simulink model "model"  (R2014a)
(part 2 of 2)

      settings: AttributesFormatString=|
      | %<ID>
      | %<Vbase>V
      | %<VLF>pu
      | %<angleLF>deg.
      | %<Name>
  bus68 : powerlib/Measurements/Load Flow Bus  LConnTagsString=a  ID=bus68  Vbase=345000  Vref=1  Vangle=0  VLF=1  angleLF=0
      settings: AttributesFormatString=|
      | %<ID>
      | %<Vbase>V
      | %<VLF>pu
      | %<angleLF>deg.
      | %<Name>
  bus69 : powerlib/Measurements/Load Flow Bus  LConnTagsString=a  ID=bus69  Vbase=345000  Vref=1  Vangle=0  VLF=1  angleLF=0
      settings: AttributesFormatString=|
      | %<ID>
      | %<Vbase>V
      | %<VLF>pu
      | %<angleLF>deg.
      | %<Name>
  bus7 : powerlib/Measurements/Load Flow Bus  LConnTagsString=a  ID=bus7  Vbase=154000  Vref=1  Vangle=0  VLF=1  angleLF=0
      settings: AttributesFormatString=|
      | %<ID>
      | %<Vbase>V
      | %<VLF>pu
      | %<angleLF>deg.
      | %<Name>
  bus70 : powerlib/Measurements/Load Flow Bus  LConnTagsString=a  ID=bus70  Vbase=345000  Vref=1  Vangle=0  VLF=1  angleLF=0
      settings: AttributesFormatString=|
      | %<ID>
      | %<Vbase>V
      | %<VLF>pu
      | %<angleLF>deg.
      | %<Name>
  bus71 : powerlib/Measurements/Load Flow Bus  LConnTagsString=a  ID=bus71  Vbase=345000  Vref=1  Vangle=0  VLF=1  angleLF=0
      settings: AttributesFormatString=|
      | %<ID>
      | %<Vbase>V
      | %<VLF>pu
      | %<angleLF>deg.
      | %<Name>
  bus72 : powerlib/Measurements/Load Flow Bus  LConnTagsString=a  ID=bus72  Vbase=345000  Vref=1  Vangle=0  VLF=1  angleLF=0
      settings: AttributesFormatString=|
      | %<ID>
      | %<Vbase>V
      | %<VLF>pu
      | %<angleLF>deg.
      | %<Name>
  bus73 : powerlib/Measurements/Load Flow Bus  LConnTagsString=a  ID=bus73  Vbase=345000  Vref=1  Vangle=0  VLF=1  angleLF=0
      settings: AttributesFormatString=|
      | %<ID>
      | %<Vbase>V
      | %<VLF>pu
      | %<angleLF>deg.
      | %<Name>
  bus74 : powerlib/Measurements/Load Flow Bus  LConnTagsString=a  ID=bus74  Vbase=345000  Vref=1  Vangle=0  VLF=1  angleLF=0
      settings: AttributesFormatString=|
      | %<ID>
      | %<Vbase>V
      | %<VLF>pu
      | %<angleLF>deg.
      | %<Name>
  bus75 : powerlib/Measurements/Load Flow Bus  LConnTagsString=a  ID=bus75  Vbase=345000  Vref=1  Vangle=0  VLF=1  angleLF=0
      settings: AttributesFormatString=|
      | %<ID>
      | %<Vbase>V
      | %<VLF>pu
      | %<angleLF>deg.
      | %<Name>
  bus76 : powerlib/Measurements/Load Flow Bus  LConnTagsString=a  ID=bus76  Vbase=345000  Vref=1  Vangle=0  VLF=1  angleLF=0
      settings: AttributesFormatString=|
      | %<ID>
      | %<Vbase>V
      | %<VLF>pu
      | %<angleLF>deg.
      | %<Name>
  bus77 : powerlib/Measurements/Load Flow Bus  LConnTagsString=a  ID=bus77  Vbase=345000  Vref=1  Vangle=0  VLF=1  angleLF=0
      settings: AttributesFormatString=|
      | %<ID>
      | %<Vbase>V
      | %<VLF>pu
      | %<angleLF>deg.
      | %<Name>
  bus78 : powerlib/Measurements/Load Flow Bus  LConnTagsString=a  ID=bus78  Vbase=345000  Vref=1  Vangle=0  VLF=1  angleLF=0
      settings: AttributesFormatString=|
      | %<ID>
      | %<Vbase>V
      | %<VLF>pu
      | %<angleLF>deg.
      | %<Name>
  bus79 : powerlib/Measurements/Load Flow Bus  LConnTagsString=a  ID=bus79  Vbase=345000  Vref=1  Vangle=0  VLF=1  angleLF=0
      settings: AttributesFormatString=|
      | %<ID>
      | %<Vbase>V
      | %<VLF>pu
      | %<angleLF>deg.
      | %<Name>
  bus8 : powerlib/Measurements/Load Flow Bus  LConnTagsString=a  ID=bus8  Vbase=154000  Vref=1  Vangle=0  VLF=1  angleLF=0
      settings: AttributesFormatString=|
      | %<ID>
      | %<Vbase>V
      | %<VLF>pu
      | %<angleLF>deg.
      | %<Name>
  bus80 : powerlib/Measurements/Load Flow Bus  LConnTagsString=a  ID=bus80  Vbase=345000  Vref=1  Vangle=0  VLF=1  angleLF=0
      settings: AttributesFormatString=|
      | %<ID>
      | %<Vbase>V
      | %<VLF>pu
      | %<angleLF>deg.
      | %<Name>
  bus81 : powerlib/Measurements/Load Flow Bus  LConnTagsString=a  ID=bus81  Vbase=345000  Vref=1  Vangle=0  VLF=1  angleLF=0
      settings: AttributesFormatString=|
      | %<ID>
      | %<Vbase>V
      | %<VLF>pu
      | %<angleLF>deg.
      | %<Name>
  bus82 : powerlib/Measurements/Load Flow Bus  LConnTagsString=a  ID=bus82  Vbase=345000  Vref=1  Vangle=0  VLF=1  angleLF=0
      settings: AttributesFormatString=|
      | %<ID>
      | %<Vbase>V
      | %<VLF>pu
      | %<angleLF>deg.
      | %<Name>
  bus83 : powerlib/Measurements/Load Flow Bus  LConnTagsString=a  ID=bus83  Vbase=345000  Vref=1  Vangle=0  VLF=1  angleLF=0
      settings: AttributesFormatString=|
      | %<ID>
      | %<Vbase>V
      | %<VLF>pu
      | %<angleLF>deg.
      | %<Name>
  bus84 : powerlib/Measurements/Load Flow Bus  LConnTagsString=a  ID=bus84  Vbase=345000  Vref=1  Vangle=0  VLF=1  angleLF=0
      settings: AttributesFormatString=|
      | %<ID>
      | %<Vbase>V
      | %<VLF>pu
      | %<angleLF>deg.
      | %<Name>
  bus85 : powerlib/Measurements/Load Flow Bus  LConnTagsString=a  ID=bus85  Vbase=345000  Vref=1  Vangle=0  VLF=1  angleLF=0
      settings: AttributesFormatString=|
      | %<ID>
      | %<Vbase>V
      | %<VLF>pu
      | %<angleLF>deg.
      | %<Name>
  bus86 : powerlib/Measurements/Load Flow Bus  LConnTagsString=a  ID=bus86  Vbase=345000  Vref=1  Vangle=0  VLF=1  angleLF=0
      settings: AttributesFormatString=|
      | %<ID>
      | %<Vbase>V
      | %<VLF>pu
      | %<angleLF>deg.
      | %<Name>
  bus87 : powerlib/Measurements/Load Flow Bus  LConnTagsString=a  ID=bus87  Vbase=345000  Vref=1  Vangle=0  VLF=1  angleLF=0
      settings: AttributesFormatString=|
      | %<ID>
      | %<Vbase>V
      | %<VLF>pu
      | %<angleLF>deg.
      | %<Name>
  bus88 : powerlib/Measurements/Load Flow Bus  LConnTagsString=a  ID=bus88  Vbase=345000  Vref=1  Vangle=0  VLF=1  angleLF=0
      settings: AttributesFormatString=|
      | %<ID>
      | %<Vbase>V
      | %<VLF>pu
      | %<angleLF>deg.
      | %<Name>
  bus89 : powerlib/Measurements/Load Flow Bus  LConnTagsString=a  ID=bus89  Vbase=345000  Vref=1  Vangle=0  VLF=1  angleLF=0
      settings: AttributesFormatString=|
      | %<ID>
      | %<Vbase>V
      | %<VLF>pu
      | %<angleLF>deg.
      | %<Name>
  bus9 : powerlib/Measurements/Load Flow Bus  LConnTagsString=a  ID=bus9  Vbase=154000  Vref=1  Vangle=0  VLF=1  angleLF=0
      settings: AttributesFormatString=|
      | %<ID>
      | %<Vbase>V
      | %<VLF>pu
      | %<angleLF>deg.
      | %<Name>
  bus90 : powerlib/Measurements/Load Flow Bus  LConnTagsString=a  ID=bus90  Vbase=345000  Vref=1  Vangle=0  VLF=1  angleLF=0
      settings: AttributesFormatString=|
      | %<ID>
      | %<Vbase>V
      | %<VLF>pu
      | %<angleLF>deg.
      | %<Name>
  bus91 : powerlib/Measurements/Load Flow Bus  LConnTagsString=a  ID=bus91  Vbase=345000  Vref=1  Vangle=0  VLF=1  angleLF=0
      settings: AttributesFormatString=|
      | %<ID>
      | %<Vbase>V
      | %<VLF>pu
      | %<angleLF>deg.
      | %<Name>
  bus92 : powerlib/Measurements/Load Flow Bus  LConnTagsString=a  ID=bus92  Vbase=345000  Vref=1  Vangle=0  VLF=1  angleLF=0
      settings: AttributesFormatString=|
      | %<ID>
      | %<Vbase>V
      | %<VLF>pu
      | %<angleLF>deg.
      | %<Name>
  bus93 : powerlib/Measurements/Load Flow Bus  LConnTagsString=a  ID=bus93  Vbase=345000  Vref=1  Vangle=0  VLF=1  angleLF=0
      settings: AttributesFormatString=|
      | %<ID>
      | %<Vbase>V
      | %<VLF>pu
      | %<angleLF>deg.
      | %<Name>
  bus94 : powerlib/Measurements/Load Flow Bus  LConnTagsString=a  ID=bus94  Vbase=345000  Vref=1  Vangle=0  VLF=1  angleLF=0
      settings: AttributesFormatString=|
      | %<ID>
      | %<Vbase>V
      | %<VLF>pu
      | %<angleLF>deg.
      | %<Name>
  bus95 : powerlib/Measurements/Load Flow Bus  LConnTagsString=a  ID=bus95  Vbase=345000  Vref=1  Vangle=0  VLF=1  angleLF=0
      settings: AttributesFormatString=|
      | %<ID>
      | %<Vbase>V
      | %<VLF>pu
      | %<angleLF>deg.
      | %<Name>
  bus96 : powerlib/Measurements/Load Flow Bus  LConnTagsString=a  ID=bus96  Vbase=345000  Vref=1  Vangle=0  VLF=1  angleLF=0
      settings: AttributesFormatString=|
      | %<ID>
      | %<Vbase>V
      | %<VLF>pu
      | %<angleLF>deg.
      | %<Name>
  bus97 : powerlib/Measurements/Load Flow Bus  LConnTagsString=a  ID=bus97  Vbase=345000  Vref=1  Vangle=0  VLF=1  angleLF=0
      settings: AttributesFormatString=|
      | %<ID>
      | %<Vbase>V
      | %<VLF>pu
      | %<angleLF>deg.
      | %<Name>
  bus98 : powerlib/Measurements/Load Flow Bus  LConnTagsString=a  ID=bus98  Vbase=345000  Vref=1  Vangle=0  VLF=1  angleLF=0
      settings: AttributesFormatString=|
      | %<ID>
      | %<Vbase>V
      | %<VLF>pu
      | %<angleLF>deg.
      | %<Name>
  bus99 : powerlib/Measurements/Load Flow Bus  LConnTagsString=a  ID=bus99  Vbase=345000  Vref=1  Vangle=0  VLF=1  angleLF=0
      settings: AttributesFormatString=|
      | %<ID>
      | %<Vbase>V
      | %<VLF>pu
      | %<angleLF>deg.
      | %<Name>
  powergui : powerlib/powergui  Priority=1  SimulationMode=Continuous  SolverType=Tustin  SampleTime=50e-6  frequency=60  SPID=off  DisableSnubberDevices=off  DisableRonSwitches=off  DisableVfSwitches=off  SwTol=0  Interpol=off  DisplayEquations=off  Ts=0  methode=off  frequencyindice=60  Pbase=100e6  ErrMax=1e-4  Iterations=50  UnitsV=kV  UnitsW=MW  FunctionMessages=off  echomessages=off  HookPort=off  EnableUseOfTLC=off  x0status=blocks  RestoreLinks=warning  ResistiveCurrentMeasurement=off  Frange=[0:2:500]  Ylog=off  Xlog=on  ShowGrid=off  save=off  variable=ZData  structure=0  ZoomFFT=off  StartTime=0.0  cycles=1  DisplayStyle=1  fundamental=60  FreqAxis=off  MaxFrequency=1000  frequencyindicesteady=1  RmsSteady=1  display=off
  connections:
  T_172009221_154000_/LConn1 -- _CN_172009221_154000_CN_119180549_154000/LConn1
  T_172009221_154000_/LConn2 -- _CN_172009221_154000_CN_119180549_154000/LConn2
  _CN_172009221_154000_CN_119180549_154000/LConn3 -- T_172009221_154000_/LConn3 -- bus1/LConn1
  T_119180549__/LConn1 -- _CN_172009221_154000_CN_119180549_154000/RConn1
  T_119180549__/LConn2 -- _CN_172009221_154000_CN_119180549_154000/RConn2
  _CN_172009221_154000_CN_119180549_154000/RConn3 -- T_119180549__/LConn3 -- bus2/LConn1
  _CN_310266400_154000_CN_312375473_154000/LConn1 -- T_310266400_345000_/RConn1 -- _CN_310266400_154000_CN_313654649_154000/LConn1 -- L_310266400/LConn1
  _CN_310266400_154000_CN_312375473_154000/LConn2 -- T_310266400_345000_/RConn2 -- _CN_310266400_154000_CN_313654649_154000/LConn2 -- L_310266400/LConn2
  _CN_310266400_154000_CN_312375473_154000/LConn3 -- T_310266400_345000_/RConn3 -- _CN_310266400_154000_CN_313654649_154000/LConn3 -- L_310266400/LConn3 -- bus3/LConn1
  _CN_310266400_154000_CN_312375473_154000/RConn1 -- T_312375473_154000_/LConn1 -- _CN_312375473_154000_CN_312375513_154000/LConn1 -- _CN_312375473_154000_CN_312375502_154000/LConn1
  _CN_310266400_154000_CN_312375473_154000/RConn2 -- T_312375473_154000_/LConn2 -- _CN_312375473_154000_CN_312375513_154000/LConn2 -- _CN_312375473_154000_CN_312375502_154000/LConn2
  _CN_310266400_154000_CN_312375473_154000/RConn3 -- T_312375473_154000_/LConn3 -- _CN_312375473_154000_CN_312375513_154000/LConn3 -- _CN_312375473_154000_CN_312375502_154000/LConn3 -- bus4/LConn1
  T_313654649_154000_/LConn1 -- _CN_310266400_154000_CN_313654649_154000/RConn1
  T_313654649_154000_/LConn2 -- _CN_310266400_154000_CN_313654649_154000/RConn2
  _CN_310266400_154000_CN_313654649_154000/RConn3 -- T_313654649_154000_/LConn3 -- bus5/LConn1
  _CN_180075042_154000_CN_168904645_154000/LConn1 -- T_180075042_154000_/LConn1 -- _CN_180075042_154000_CN_313283373_154000/LConn1
  _CN_180075042_154000_CN_168904645_154000/LConn2 -- T_180075042_154000_/LConn2 -- _CN_180075042_154000_CN_313283373_154000/LConn2
  _CN_180075042_154000_CN_168904645_154000/LConn3 -- T_180075042_154000_/LConn3 -- _CN_180075042_154000_CN_313283373_154000/LConn3 -- bus6/LConn1
  T_168904645__양양변전소/LConn1 -- _CN_180075042_154000_CN_168904645_154000/RConn1
  T_168904645__양양변전소/LConn2 -- _CN_180075042_154000_CN_168904645_154000/RConn2
  _CN_180075042_154000_CN_168904645_154000/RConn3 -- T_168904645__양양변전소/LConn3 -- bus7/LConn1
  T_313283373_154000_/LConn1 -- _CN_180075042_154000_CN_313283373_154000/RConn1
  T_313283373_154000_/LConn2 -- _CN_180075042_154000_CN_313283373_154000/RConn2
  _CN_180075042_154000_CN_313283373_154000/RConn3 -- T_313283373_154000_/LConn3 -- bus8/LConn1
  T_311068711_154000_/LConn1 -- _CN_311068711_154000_CN_205296347_154000/LConn1
  T_311068711_154000_/LConn2 -- _CN_311068711_154000_CN_205296347_154000/LConn2
  _CN_311068711_154000_CN_205296347_154000/LConn3 -- T_311068711_154000_/LConn3 -- bus9/LConn1
  _CN_311068711_154000_CN_205296347_154000/RConn1 -- T_205296347__/LConn1 -- _CN_308953870_154000_CN_205296347_154000/LConn1
  _CN_311068711_154000_CN_205296347_154000/RConn2 -- T_205296347__/LConn2 -- _CN_308953870_154000_CN_205296347_154000/LConn2
  _CN_311068711_154000_CN_205296347_154000/RConn3 -- T_205296347__/LConn3 -- _CN_308953870_154000_CN_205296347_154000/LConn3 -- bus10/LConn1
  T_311144496_154000_/LConn1 -- _CN_311144496_154000_CN_316124722_154000/LConn1
  T_311144496_154000_/LConn2 -- _CN_311144496_154000_CN_316124722_154000/LConn2
  _CN_311144496_154000_CN_316124722_154000/LConn3 -- T_311144496_154000_/LConn3 -- bus11/LConn1
  T_316124722_154000_/LConn1 -- _CN_311144496_154000_CN_316124722_154000/RConn1
  T_316124722_154000_/LConn2 -- _CN_311144496_154000_CN_316124722_154000/RConn2
  _CN_311144496_154000_CN_316124722_154000/RConn3 -- T_316124722_154000_/LConn3 -- bus12/LConn1
  _CN_310293553_154000_CN_313388404_154000/LConn1 -- T_310293553_345000_/RConn1 -- L_310293553/LConn1
  _CN_310293553_154000_CN_313388404_154000/LConn2 -- T_310293553_345000_/RConn2 -- L_310293553/LConn2
  _CN_310293553_154000_CN_313388404_154000/LConn3 -- T_310293553_345000_/RConn3 -- L_310293553/LConn3 -- bus13/LConn1
  _CN_310293553_154000_CN_313388404_154000/RConn1 -- T_313388404_154000_/LConn1 -- _CN_313388404_154000_CN_313388489_154000/LConn1
  _CN_310293553_154000_CN_313388404_154000/RConn2 -- T_313388404_154000_/LConn2 -- _CN_313388404_154000_CN_313388489_154000/LConn2
  _CN_310293553_154000_CN_313388404_154000/RConn3 -- T_313388404_154000_/LConn3 -- _CN_313388404_154000_CN_313388489_154000/LConn3 -- bus14/LConn1
  T_125840986__/LConn1 -- _CN_125840986_154000_CN_126047655_154000/LConn1
  T_125840986__/LConn2 -- _CN_125840986_154000_CN_126047655_154000/LConn2
  _CN_125840986_154000_CN_126047655_154000/LConn3 -- T_125840986__/LConn3 -- bus15/LConn1
  T_126047655__/LConn1 -- _CN_125840986_154000_CN_126047655_154000/RConn1
  T_126047655__/LConn2 -- _CN_125840986_154000_CN_126047655_154000/RConn2
  _CN_125840986_154000_CN_126047655_154000/RConn3 -- T_126047655__/LConn3 -- bus16/LConn1
  T_231045732__/LConn1 -- _CN_231045732_154000_CN_310574464_154000/LConn1
  T_231045732__/LConn2 -- _CN_231045732_154000_CN_310574464_154000/LConn2
  _CN_231045732_154000_CN_310574464_154000/LConn3 -- T_231045732__/LConn3 -- bus17/LConn1
  _CN_231045732_154000_CN_310574464_154000/RConn1 -- T_310574464__신진천_(Sin_Jincheon)/RConn1 -- _CN_308953870_154000_CN_310574464_154000/LConn1 -- L_310574464/LConn1
  _CN_231045732_154000_CN_310574464_154000/RConn2 -- T_310574464__신진천_(Sin_Jincheon)/RConn2 -- _CN_308953870_154000_CN_310574464_154000/LConn2 -- L_310574464/LConn2
  _CN_231045732_154000_CN_310574464_154000/RConn3 -- T_310574464__신진천_(Sin_Jincheon)/RConn3 -- _CN_308953870_154000_CN_310574464_154000/LConn3 -- L_310574464/LConn3 -- bus18/LConn1
  _CN_312297594_154000_CN_312297600_154000/LConn1 -- T_312297594_345000_신파주_(Sin_Paju)/RConn1 -- _CN_312297594_154000_CN_310963709_154000/LConn1 -- L_312297594/LConn1
  _CN_312297594_154000_CN_312297600_154000/LConn2 -- T_312297594_345000_신파주_(Sin_Paju)/RConn2 -- _CN_312297594_154000_CN_310963709_154000/LConn2 -- L_312297594/LConn2
  _CN_312297594_154000_CN_312297600_154000/LConn3 -- T_312297594_345000_신파주_(Sin_Paju)/RConn3 -- _CN_312297594_154000_CN_310963709_154000/LConn3 -- L_312297594/LConn3 -- bus19/LConn1
  T_312297600_154000_/LConn1 -- _CN_312297594_154000_CN_312297600_154000/RConn1
  T_312297600_154000_/LConn2 -- _CN_312297594_154000_CN_312297600_154000/RConn2
  _CN_312297594_154000_CN_312297600_154000/RConn3 -- T_312297600_154000_/LConn3 -- bus20/LConn1
  _CN_312297594_154000_CN_310963709_154000/RConn1 -- T_310963709__양주_(Yangju)/RConn1 -- L_310963709/LConn1
  _CN_312297594_154000_CN_310963709_154000/RConn2 -- T_310963709__양주_(Yangju)/RConn2 -- L_310963709/LConn2
  _CN_312297594_154000_CN_310963709_154000/RConn3 -- T_310963709__양주_(Yangju)/RConn3 -- L_310963709/LConn3 -- bus21/LConn1
  T_313247877_154000_/LConn1 -- _CN_313247877_154000_CN_313264823_154000/LConn1
  T_313247877_154000_/LConn2 -- _CN_313247877_154000_CN_313264823_154000/LConn2
  _CN_313247877_154000_CN_313264823_154000/LConn3 -- T_313247877_154000_/LConn3 -- bus22/LConn1
  T_313264823_154000_/LConn1 -- _CN_313247877_154000_CN_313264823_154000/RConn1
  T_313264823_154000_/LConn2 -- _CN_313247877_154000_CN_313264823_154000/RConn2
  _CN_313247877_154000_CN_313264823_154000/RConn3 -- T_313264823_154000_/LConn3 -- bus23/LConn1
  T_297601178_154000_/LConn1 -- _CN_297601178_154000_CN_297601183_154000/LConn1
  T_297601178_154000_/LConn2 -- _CN_297601178_154000_CN_297601183_154000/LConn2
  _CN_297601178_154000_CN_297601183_154000/LConn3 -- T_297601178_154000_/LConn3 -- bus24/LConn1
  _CN_297601178_154000_CN_297601183_154000/RConn1 -- T_297601183_154000_/LConn1 -- _CN_297601183_154000_CN_308765055_154000/LConn1 -- _CN_297601183_154000_CN_308765054_154000/LConn1
  _CN_297601178_154000_CN_297601183_154000/RConn2 -- T_297601183_154000_/LConn2 -- _CN_297601183_154000_CN_308765055_154000/LConn2 -- _CN_297601183_154000_CN_308765054_154000/LConn2
  _CN_297601178_154000_CN_297601183_154000/RConn3 -- T_297601183_154000_/LConn3 -- _CN_297601183_154000_CN_308765055_154000/LConn3 -- _CN_297601183_154000_CN_308765054_154000/LConn3 -- bus25/LConn1
  _CN_297601183_154000_CN_308765055_154000/RConn1 -- T_308765055__/RConn1 -- L_308765055/LConn1
  _CN_297601183_154000_CN_308765055_154000/RConn2 -- T_308765055__/RConn2 -- L_308765055/LConn2
  _CN_297601183_154000_CN_308765055_154000/RConn3 -- T_308765055__/RConn3 -- L_308765055/LConn3 -- bus26/LConn1
  _CN_297601183_154000_CN_308765054_154000/RConn1 -- T_308765054_345000_/LConn1 -- _CN_313355118_154000_CN_308765054_154000/LConn1
  _CN_297601183_154000_CN_308765054_154000/RConn2 -- T_308765054_345000_/LConn2 -- _CN_313355118_154000_CN_308765054_154000/LConn2
  _CN_297601183_154000_CN_308765054_154000/RConn3 -- T_308765054_345000_/LConn3 -- _CN_313355118_154000_CN_308765054_154000/LConn3 -- bus27/LConn1
  _CN_310065312_154000_CN_313280968_154000/LConn1 -- T_310065312__/RConn1 -- _CN_310065312_154000_CN_312319437_154000/LConn1 -- L_310065312/LConn1
  _CN_310065312_154000_CN_313280968_154000/LConn2 -- T_310065312__/RConn2 -- _CN_310065312_154000_CN_312319437_154000/LConn2 -- L_310065312/LConn2
  _CN_310065312_154000_CN_313280968_154000/LConn3 -- T_310065312__/RConn3 -- _CN_310065312_154000_CN_312319437_154000/LConn3 -- L_310065312/LConn3 -- bus28/LConn1
  T_313280968_154000_/LConn1 -- _CN_310065312_154000_CN_313280968_154000/RConn1
  T_313280968_154000_/LConn2 -- _CN_310065312_154000_CN_313280968_154000/RConn2
  _CN_310065312_154000_CN_313280968_154000/RConn3 -- T_313280968_154000_/LConn3 -- bus29/LConn1
  T_312319437_154000_/LConn1 -- _CN_310065312_154000_CN_312319437_154000/RConn1
  T_312319437_154000_/LConn2 -- _CN_310065312_154000_CN_312319437_154000/RConn2
  _CN_310065312_154000_CN_312319437_154000/RConn3 -- T_312319437_154000_/LConn3 -- bus30/LConn1
  _CN_310421552_154000_CN_312319401_154000/LConn1 -- T_310421552__/RConn1 -- _CN_310421552_154000_CN_312319351_154000/LConn1 -- L_310421552/LConn1
  _CN_310421552_154000_CN_312319401_154000/LConn2 -- T_310421552__/RConn2 -- _CN_310421552_154000_CN_312319351_154000/LConn2 -- L_310421552/LConn2
  _CN_310421552_154000_CN_312319401_154000/LConn3 -- T_310421552__/RConn3 -- _CN_310421552_154000_CN_312319351_154000/LConn3 -- L_310421552/LConn3 -- bus31/LConn1
  T_312319401__/LConn1 -- _CN_310421552_154000_CN_312319401_154000/RConn1
  T_312319401__/LConn2 -- _CN_310421552_154000_CN_312319401_154000/RConn2
  _CN_310421552_154000_CN_312319401_154000/RConn3 -- T_312319401__/LConn3 -- bus32/LConn1
  T_312319351_154000_/LConn1 -- _CN_310421552_154000_CN_312319351_154000/RConn1
  T_312319351_154000_/LConn2 -- _CN_310421552_154000_CN_312319351_154000/RConn2
  _CN_310421552_154000_CN_312319351_154000/RConn3 -- T_312319351_154000_/LConn3 -- bus33/LConn1
  _CN_312375473_154000_CN_312375513_154000/RConn1 -- T_312375513_154000_/LConn1 -- _CN_312375513_154000_CN_312375515_154000/LConn1 -- _CN_312375513_154000_CN_308770040_154000/LConn1
  _CN_312375473_154000_CN_312375513_154000/RConn2 -- T_312375513_154000_/LConn2 -- _CN_312375513_154000_CN_312375515_154000/LConn2 -- _CN_312375513_154000_CN_308770040_154000/LConn2
  _CN_312375473_154000_CN_312375513_154000/RConn3 -- T_312375513_154000_/LConn3 -- _CN_312375513_154000_CN_312375515_154000/LConn3 -- _CN_312375513_154000_CN_308770040_154000/LConn3 -- bus34/LConn1
  T_312375502_154000_/LConn1 -- _CN_312375473_154000_CN_312375502_154000/RConn1
  T_312375502_154000_/LConn2 -- _CN_312375473_154000_CN_312375502_154000/RConn2
  _CN_312375473_154000_CN_312375502_154000/RConn3 -- T_312375502_154000_/LConn3 -- bus35/LConn1
  _CN_313264824_154000_CN_308953870_154000/LConn1 -- T_313264824_154000_/LConn1 -- _CN_313264824_154000_CN_371952375_154000/LConn1
  _CN_313264824_154000_CN_308953870_154000/LConn2 -- T_313264824_154000_/LConn2 -- _CN_313264824_154000_CN_371952375_154000/LConn2
  _CN_313264824_154000_CN_308953870_154000/LConn3 -- T_313264824_154000_/LConn3 -- _CN_313264824_154000_CN_371952375_154000/LConn3 -- bus36/LConn1
  _CN_313264824_154000_CN_308953870_154000/RConn1 -- T_308953870__신진천_(Sin_Jincheon)/LConn1 -- _CN_308953870_154000_CN_310574464_154000/RConn1 -- _CN_308953870_154000_CN_205296347_154000/RConn1
  _CN_313264824_154000_CN_308953870_154000/RConn2 -- T_308953870__신진천_(Sin_Jincheon)/LConn2 -- _CN_308953870_154000_CN_310574464_154000/RConn2 -- _CN_308953870_154000_CN_205296347_154000/RConn2
  _CN_313264824_154000_CN_308953870_154000/RConn3 -- T_308953870__신진천_(Sin_Jincheon)/LConn3 -- _CN_308953870_154000_CN_310574464_154000/RConn3 -- _CN_308953870_154000_CN_205296347_154000/RConn3 -- bus37/LConn1
  T_371952375__/LConn1 -- _CN_313264824_154000_CN_371952375_154000/RConn1
  T_371952375__/LConn2 -- _CN_313264824_154000_CN_371952375_154000/RConn2
  _CN_313264824_154000_CN_371952375_154000/RConn3 -- T_371952375__/LConn3 -- bus38/LConn1
  T_372869919_154000_/LConn1 -- _CN_372869919_154000_CN_310226151_154000/LConn1
  T_372869919_154000_/LConn2 -- _CN_372869919_154000_CN_310226151_154000/LConn2
  _CN_372869919_154000_CN_310226151_154000/LConn3 -- T_372869919_154000_/LConn3 -- bus39/LConn1
  _CN_372869919_154000_CN_310226151_154000/RConn1 -- T_310226151_345000_신광주_(Sin_Gwangju)/RConn1 -- L_310226151/LConn1
  _CN_372869919_154000_CN_310226151_154000/RConn2 -- T_310226151_345000_신광주_(Sin_Gwangju)/RConn2 -- L_310226151/LConn2
  _CN_372869919_154000_CN_310226151_154000/RConn3 -- T_310226151_345000_신광주_(Sin_Gwangju)/RConn3 -- L_310226151/LConn3 -- bus40/LConn1
  _CN_312375499_154000_CN_312375501_154000/LConn1 -- T_312375499_154000_/LConn1 -- _CN_312375499_154000_CN_308770040_154000/LConn1
  _CN_312375499_154000_CN_312375501_154000/LConn2 -- T_312375499_154000_/LConn2 -- _CN_312375499_154000_CN_308770040_154000/LConn2
  _CN_312375499_154000_CN_312375501_154000/LConn3 -- T_312375499_154000_/LConn3 -- _CN_312375499_154000_CN_308770040_154000/LConn3 -- bus41/LConn1
  T_312375501_154000_/LConn1 -- _CN_312375499_154000_CN_312375501_154000/RConn1
  T_312375501_154000_/LConn2 -- _CN_312375499_154000_CN_312375501_154000/RConn2
  _CN_312375499_154000_CN_312375501_154000/RConn3 -- T_312375501_154000_/LConn3 -- bus42/LConn1
  _CN_312375499_154000_CN_308770040_154000/RConn1 -- T_308770040__고령_(Goryeong)/RConn1 -- _CN_312375513_154000_CN_308770040_154000/RConn1 -- L_308770040/LConn1
  _CN_312375499_154000_CN_308770040_154000/RConn2 -- T_308770040__고령_(Goryeong)/RConn2 -- _CN_312375513_154000_CN_308770040_154000/RConn2 -- L_308770040/LConn2
  _CN_312375499_154000_CN_308770040_154000/RConn3 -- T_308770040__고령_(Goryeong)/RConn3 -- _CN_312375513_154000_CN_308770040_154000/RConn3 -- L_308770040/LConn3 -- bus43/LConn1
  _CN_310395601_154000_CN_310395617_154000/LConn1 -- T_310395601_154000_/LConn1 -- _CN_310395601_154000_CN_310281776_154000/LConn1
  _CN_310395601_154000_CN_310395617_154000/LConn2 -- T_310395601_154000_/LConn2 -- _CN_310395601_154000_CN_310281776_154000/LConn2
  _CN_310395601_154000_CN_310395617_154000/LConn3 -- T_310395601_154000_/LConn3 -- _CN_310395601_154000_CN_310281776_154000/LConn3 -- bus44/LConn1
  T_310395617_154000_/LConn1 -- _CN_310395601_154000_CN_310395617_154000/RConn1
  T_310395617_154000_/LConn2 -- _CN_310395601_154000_CN_310395617_154000/RConn2
  _CN_310395601_154000_CN_310395617_154000/RConn3 -- T_310395617_154000_/LConn3 -- bus45/LConn1
  _CN_310395601_154000_CN_310281776_154000/RConn1 -- T_310281776_345000_신김해_(Sin_Gimhae)/RConn1 -- _CN_415837596_154000_CN_310281776_154000/LConn1 -- L_310281776/LConn1
  _CN_310395601_154000_CN_310281776_154000/RConn2 -- T_310281776_345000_신김해_(Sin_Gimhae)/RConn2 -- _CN_415837596_154000_CN_310281776_154000/LConn2 -- L_310281776/LConn2
  _CN_310395601_154000_CN_310281776_154000/RConn3 -- T_310281776_345000_신김해_(Sin_Gimhae)/RConn3 -- _CN_415837596_154000_CN_310281776_154000/LConn3 -- L_310281776/LConn3 -- bus46/LConn1
  T_312375515_154000_/LConn1 -- _CN_312375513_154000_CN_312375515_154000/RConn1
  T_312375515_154000_/LConn2 -- _CN_312375513_154000_CN_312375515_154000/RConn2
  _CN_312375513_154000_CN_312375515_154000/RConn3 -- T_312375515_154000_/LConn3 -- bus47/LConn1
  _CN_143609113_154000_CN_312424737_154000/LConn1 -- T_143609113_345000_/RConn1 -- L_143609113/LConn1
  _CN_143609113_154000_CN_312424737_154000/LConn2 -- T_143609113_345000_/RConn2 -- L_143609113/LConn2
  _CN_143609113_154000_CN_312424737_154000/LConn3 -- T_143609113_345000_/RConn3 -- L_143609113/LConn3 -- bus48/LConn1
  _CN_143609113_154000_CN_312424737_154000/RConn1 -- T_312424737_154000_/LConn1 -- _CN_312424737_154000_CN_313355100_154000/LConn1
  _CN_143609113_154000_CN_312424737_154000/RConn2 -- T_312424737_154000_/LConn2 -- _CN_312424737_154000_CN_313355100_154000/LConn2
  _CN_143609113_154000_CN_312424737_154000/RConn3 -- T_312424737_154000_/LConn3 -- _CN_312424737_154000_CN_313355100_154000/LConn3 -- bus49/LConn1
  T_312424733_154000_/LConn1 -- _CN_312424733_154000_CN_312424741_154000/LConn1
  T_312424733_154000_/LConn2 -- _CN_312424733_154000_CN_312424741_154000/LConn2
  _CN_312424733_154000_CN_312424741_154000/LConn3 -- T_312424733_154000_/LConn3 -- bus50/LConn1
  T_312424741_154000_/LConn1 -- _CN_312424733_154000_CN_312424741_154000/RConn1
  T_312424741_154000_/LConn2 -- _CN_312424733_154000_CN_312424741_154000/RConn2
  _CN_312424733_154000_CN_312424741_154000/RConn3 -- T_312424741_154000_/LConn3 -- bus51/LConn1
  T_313355100_154000_/LConn1 -- _CN_312424737_154000_CN_313355100_154000/RConn1
  T_313355100_154000_/LConn2 -- _CN_312424737_154000_CN_313355100_154000/RConn2
  _CN_312424737_154000_CN_313355100_154000/RConn3 -- T_313355100_154000_/LConn3 -- bus52/LConn1
  _CN_313355118_154000_CN_313355123_154000/LConn1 -- T_313355118_154000_/LConn1 -- _CN_313355118_154000_CN_308765054_154000/RConn1
  _CN_313355118_154000_CN_313355123_154000/LConn2 -- T_313355118_154000_/LConn2 -- _CN_313355118_154000_CN_308765054_154000/RConn2
  _CN_313355118_154000_CN_313355123_154000/LConn3 -- T_313355118_154000_/LConn3 -- _CN_313355118_154000_CN_308765054_154000/RConn3 -- bus53/LConn1
  T_313355123_154000_/LConn1 -- _CN_313355118_154000_CN_313355123_154000/RConn1
  T_313355123_154000_/LConn2 -- _CN_313355118_154000_CN_313355123_154000/RConn2
  _CN_313355118_154000_CN_313355123_154000/RConn3 -- T_313355123_154000_/LConn3 -- bus54/LConn1
  T_313388489_154000_/LConn1 -- _CN_313388404_154000_CN_313388489_154000/RConn1
  T_313388489_154000_/LConn2 -- _CN_313388404_154000_CN_313388489_154000/RConn2
  _CN_313388404_154000_CN_313388489_154000/RConn3 -- T_313388489_154000_/LConn3 -- bus55/LConn1
  T_312408983_154000_/LConn1 -- _CN_312408983_154000_CN_235152925_154000/LConn1
  T_312408983_154000_/LConn2 -- _CN_312408983_154000_CN_235152925_154000/LConn2
  _CN_312408983_154000_CN_235152925_154000/LConn3 -- T_312408983_154000_/LConn3 -- bus56/LConn1
  G_235152925_인천발전소/RConn1 -- _CN_312408983_154000_CN_235152925_154000/RConn1
  G_235152925_인천발전소/RConn2 -- _CN_312408983_154000_CN_235152925_154000/RConn2
  _CN_312408983_154000_CN_235152925_154000/RConn3 -- G_235152925_인천발전소/RConn3 -- bus57/LConn1
  T_415837596__/LConn1 -- _CN_415837596_154000_CN_310281776_154000/RConn1
  T_415837596__/LConn2 -- _CN_415837596_154000_CN_310281776_154000/RConn2
  _CN_415837596_154000_CN_310281776_154000/RConn3 -- T_415837596__/LConn3 -- bus58/LConn1
  T_312319393_154000_/LConn1 -- _CN_312319393_154000_CN_308711344_154000/LConn1
  T_312319393_154000_/LConn2 -- _CN_312319393_154000_CN_308711344_154000/LConn2
  _CN_312319393_154000_CN_308711344_154000/LConn3 -- T_312319393_154000_/LConn3 -- bus59/LConn1
  _CN_312319393_154000_CN_308711344_154000/RConn1 -- T_308711344_345000_서서울_(Seo_Seoul)/RConn1 -- L_308711344/LConn1
  _CN_312319393_154000_CN_308711344_154000/RConn2 -- T_308711344_345000_서서울_(Seo_Seoul)/RConn2 -- L_308711344/LConn2
  _CN_312319393_154000_CN_308711344_154000/RConn3 -- T_308711344_345000_서서울_(Seo_Seoul)/RConn3 -- L_308711344/LConn3 -- bus60/LConn1
  _CN_310574464_345000_CN_310065312_345000/LConn1 -- T_310574464__신진천_(Sin_Jincheon)/LConn1 -- _CN_310574464_345000_CN_308953834_345000/LConn1
  _CN_310574464_345000_CN_310065312_345000/LConn2 -- T_310574464__신진천_(Sin_Jincheon)/LConn2 -- _CN_310574464_345000_CN_308953834_345000/LConn2
  _CN_310574464_345000_CN_310065312_345000/LConn3 -- T_310574464__신진천_(Sin_Jincheon)/LConn3 -- _CN_310574464_345000_CN_308953834_345000/LConn3 -- bus61/LConn1
  _CN_310574464_345000_CN_310065312_345000/RConn1 -- T_310065312__/LConn1 -- _CN_310065312_345000_CN_156580308_345000/LConn1
  _CN_310574464_345000_CN_310065312_345000/RConn2 -- T_310065312__/LConn2 -- _CN_310065312_345000_CN_156580308_345000/LConn2
  _CN_310574464_345000_CN_310065312_345000/RConn3 -- T_310065312__/LConn3 -- _CN_310065312_345000_CN_156580308_345000/LConn3 -- bus62/LConn1
  _CN_310574464_345000_CN_308953834_345000/RConn1 -- T_308953834_345000_/LConn1 -- _CN_308953834_345000_CN_313247875_345000/LConn1
  _CN_310574464_345000_CN_308953834_345000/RConn2 -- T_308953834_345000_/LConn2 -- _CN_308953834_345000_CN_313247875_345000/LConn2
  _CN_310574464_345000_CN_308953834_345000/RConn3 -- T_308953834_345000_/LConn3 -- _CN_308953834_345000_CN_313247875_345000/LConn3 -- bus63/LConn1
  T_310574466_345000_/LConn1 -- _CN_310574466_345000_CN_143756950_345000/LConn1
  T_310574466_345000_/LConn2 -- _CN_310574466_345000_CN_143756950_345000/LConn2
  _CN_310574466_345000_CN_143756950_345000/LConn3 -- T_310574466_345000_/LConn3 -- bus64/LConn1
  _CN_310574466_345000_CN_143756950_345000/RConn1 -- T_143756950_345000_/LConn1 -- _CN_143756950_345000_CN_143609113_345000/LConn1
  _CN_310574466_345000_CN_143756950_345000/RConn2 -- T_143756950_345000_/LConn2 -- _CN_143756950_345000_CN_143609113_345000/LConn2
  _CN_310574466_345000_CN_143756950_345000/RConn3 -- T_143756950_345000_/LConn3 -- _CN_143756950_345000_CN_143609113_345000/LConn3 -- bus65/LConn1
  _CN_117614725_345000_CN_310266400_345000/LConn1 -- T_117614725__/LConn1 -- _CN_117614725_345000_CN_310281776_345000/LConn1
  _CN_117614725_345000_CN_310266400_345000/LConn2 -- T_117614725__/LConn2 -- _CN_117614725_345000_CN_310281776_345000/LConn2
  _CN_117614725_345000_CN_310266400_345000/LConn3 -- T_117614725__/LConn3 -- _CN_117614725_345000_CN_310281776_345000/LConn3 -- bus66/LConn1
  _CN_117614725_345000_CN_310266400_345000/RConn1 -- T_310266400_345000_/LConn1 -- _CN_310266398_345000_CN_310266400_345000/LConn1
  _CN_117614725_345000_CN_310266400_345000/RConn2 -- T_310266400_345000_/LConn2 -- _CN_310266398_345000_CN_310266400_345000/LConn2
  _CN_117614725_345000_CN_310266400_345000/RConn3 -- T_310266400_345000_/LConn3 -- _CN_310266398_345000_CN_310266400_345000/LConn3 -- bus67/LConn1
  T_310281776_345000_신김해_(Sin_Gimhae)/LConn1 -- _CN_117614725_345000_CN_310281776_345000/RConn1
  T_310281776_345000_신김해_(Sin_Gimhae)/LConn2 -- _CN_117614725_345000_CN_310281776_345000/RConn2
  _CN_117614725_345000_CN_310281776_345000/RConn3 -- T_310281776_345000_신김해_(Sin_Gimhae)/LConn3 -- bus68/LConn1
  T_310281736_345000_/LConn1 -- _CN_310281736_345000_CN_143987473_345000/LConn1
  T_310281736_345000_/LConn2 -- _CN_310281736_345000_CN_143987473_345000/LConn2
  _CN_310281736_345000_CN_143987473_345000/LConn3 -- T_310281736_345000_/LConn3 -- bus69/LConn1
  _CN_310281736_345000_CN_143987473_345000/RConn1 -- T_143987473_345000_/LConn1 -- _CN_143987473_345000_CN_143605191_345000/LConn1 -- _CN_143987473_345000_CN_403402683_345000/LConn1
  _CN_310281736_345000_CN_143987473_345000/RConn2 -- T_143987473_345000_/LConn2 -- _CN_143987473_345000_CN_143605191_345000/LConn2 -- _CN_143987473_345000_CN_403402683_345000/LConn2
  _CN_310281736_345000_CN_143987473_345000/RConn3 -- T_143987473_345000_/LConn3 -- _CN_143987473_345000_CN_143605191_345000/LConn3 -- _CN_143987473_345000_CN_403402683_345000/LConn3 -- bus70/LConn1
  T_310943500_345000_동서울_변전소/LConn1 -- _CN_310943500_345000_CN_310961238_345000/LConn1
  T_310943500_345000_동서울_변전소/LConn2 -- _CN_310943500_345000_CN_310961238_345000/LConn2
  _CN_310943500_345000_CN_310961238_345000/LConn3 -- T_310943500_345000_동서울_변전소/LConn3 -- bus71/LConn1
  _CN_310943500_345000_CN_310961238_345000/RConn1 -- T_310961238_345000_/LConn1 -- _CN_310961238_345000_CN_310963709_345000/LConn1
  _CN_310943500_345000_CN_310961238_345000/RConn2 -- T_310961238_345000_/LConn2 -- _CN_310961238_345000_CN_310963709_345000/LConn2
  _CN_310943500_345000_CN_310961238_345000/RConn3 -- T_310961238_345000_/LConn3 -- _CN_310961238_345000_CN_310963709_345000/LConn3 -- bus72/LConn1
  _CN_143987473_345000_CN_143605191_345000/RConn1 -- T_143605191_345000_신포항_(Sin_Pohang)/LConn1 -- _CN_310995902_345000_CN_143605191_345000/LConn1 -- _CN_143605191_345000_CN_403402683_345000/LConn1 -- _CN_143605191_345000_CN_156580308_345000/LConn1
  _CN_143987473_345000_CN_143605191_345000/RConn2 -- T_143605191_345000_신포항_(Sin_Pohang)/LConn2 -- _CN_310995902_345000_CN_143605191_345000/LConn2 -- _CN_143605191_345000_CN_403402683_345000/LConn2 -- _CN_143605191_345000_CN_156580308_345000/LConn2
  _CN_143987473_345000_CN_143605191_345000/RConn3 -- T_143605191_345000_신포항_(Sin_Pohang)/LConn3 -- _CN_310995902_345000_CN_143605191_345000/LConn3 -- _CN_143605191_345000_CN_403402683_345000/LConn3 -- _CN_143605191_345000_CN_156580308_345000/LConn3 -- bus73/LConn1
  _CN_143987473_345000_CN_403402683_345000/RConn1 -- G_403402683_Wolsung_Nuclear_Power_Station/RConn1 -- _CN_143609113_345000_CN_403402683_345000/LConn1 -- _CN_143605191_345000_CN_403402683_345000/RConn1
  _CN_143987473_345000_CN_403402683_345000/RConn2 -- G_403402683_Wolsung_Nuclear_Power_Station/RConn2 -- _CN_143609113_345000_CN_403402683_345000/LConn2 -- _CN_143605191_345000_CN_403402683_345000/RConn2
  _CN_143987473_345000_CN_403402683_345000/RConn3 -- G_403402683_Wolsung_Nuclear_Power_Station/RConn3 -- _CN_143609113_345000_CN_403402683_345000/LConn3 -- _CN_143605191_345000_CN_403402683_345000/RConn3 -- bus74/LConn1
  _CN_143756950_345000_CN_143609113_345000/RConn1 -- T_143609113_345000_/LConn1 -- _CN_143609113_345000_CN_308765055_345000/LConn1 -- _CN_143609113_345000_CN_403402683_345000/RConn1
  _CN_143756950_345000_CN_143609113_345000/RConn2 -- T_143609113_345000_/LConn2 -- _CN_143609113_345000_CN_308765055_345000/LConn2 -- _CN_143609113_345000_CN_403402683_345000/RConn2
  _CN_143756950_345000_CN_143609113_345000/RConn3 -- T_143609113_345000_/LConn3 -- _CN_143609113_345000_CN_308765055_345000/LConn3 -- bus75/LConn1 -- _CN_143609113_345000_CN_403402683_345000/RConn3
  _CN_308733209_345000_CN_310247600_345000/LConn1 -- T_308733209_345000_/LConn1 -- _CN_308733209_345000_CN_308733211_345000/LConn1
  _CN_308733209_345000_CN_310247600_345000/LConn2 -- T_308733209_345000_/LConn2 -- _CN_308733209_345000_CN_308733211_345000/LConn2
  _CN_308733209_345000_CN_310247600_345000/LConn3 -- T_308733209_345000_/LConn3 -- _CN_308733209_345000_CN_308733211_345000/LConn3 -- bus76/LConn1
  _CN_308733209_345000_CN_310247600_345000/RConn1 -- T_310247600_345000_/LConn1 -- _CN_310247600_345000_CN_310247604_345000/LConn1
  _CN_308733209_345000_CN_310247600_345000/RConn2 -- T_310247600_345000_/LConn2 -- _CN_310247600_345000_CN_310247604_345000/LConn2
  _CN_308733209_345000_CN_310247600_345000/RConn3 -- T_310247600_345000_/LConn3 -- _CN_310247600_345000_CN_310247604_345000/LConn3 -- bus77/LConn1
  T_308733211__/LConn1 -- _CN_308733209_345000_CN_308733211_345000/RConn1
  T_308733211__/LConn2 -- _CN_308733209_345000_CN_308733211_345000/RConn2
  _CN_308733209_345000_CN_308733211_345000/RConn3 -- T_308733211__/LConn3 -- bus78/LConn1
  T_308765055__/LConn1 -- _CN_143609113_345000_CN_308765055_345000/RConn1
  T_308765055__/LConn2 -- _CN_143609113_345000_CN_308765055_345000/RConn2
  _CN_143609113_345000_CN_308765055_345000/RConn3 -- T_308765055__/LConn3 -- bus79/LConn1
  _CN_198717854_345000_CN_307934520_345000/LConn1 -- T_198717854__/LConn1 -- _CN_198717854_345000_CN_199954117_345000/LConn1
  _CN_198717854_345000_CN_307934520_345000/LConn2 -- T_198717854__/LConn2 -- _CN_198717854_345000_CN_199954117_345000/LConn2
  _CN_198717854_345000_CN_307934520_345000/LConn3 -- T_198717854__/LConn3 -- _CN_198717854_345000_CN_199954117_345000/LConn3 -- bus80/LConn1
  _CN_198717854_345000_CN_307934520_345000/RConn1 -- T_307934520__/LConn1 -- _CN_307934520_345000_CN_310421552_345000/LConn1
  _CN_198717854_345000_CN_307934520_345000/RConn2 -- T_307934520__/LConn2 -- _CN_307934520_345000_CN_310421552_345000/LConn2
  _CN_198717854_345000_CN_307934520_345000/RConn3 -- T_307934520__/LConn3 -- _CN_307934520_345000_CN_310421552_345000/LConn3 -- bus81/LConn1
  T_199954117__/LConn1 -- _CN_198717854_345000_CN_199954117_345000/RConn1
  T_199954117__/LConn2 -- _CN_198717854_345000_CN_199954117_345000/RConn2
  _CN_198717854_345000_CN_199954117_345000/RConn3 -- T_199954117__/LConn3 -- bus82/LConn1
  _CN_310065312_345000_CN_156580308_345000/RConn1 -- T_156580308_345000_신옥천_(Sin_Okcheon)/LConn1 -- _CN_143605191_345000_CN_156580308_345000/RConn1 -- _CN_119001902_345000_CN_156580308_345000/LConn1
  _CN_310065312_345000_CN_156580308_345000/RConn2 -- T_156580308_345000_신옥천_(Sin_Okcheon)/LConn2 -- _CN_143605191_345000_CN_156580308_345000/RConn2 -- _CN_119001902_345000_CN_156580308_345000/LConn2
  _CN_310065312_345000_CN_156580308_345000/RConn3 -- T_156580308_345000_신옥천_(Sin_Okcheon)/LConn3 -- _CN_143605191_345000_CN_156580308_345000/RConn3 -- bus83/LConn1 -- _CN_119001902_345000_CN_156580308_345000/LConn3
  T_310247604__/LConn1 -- _CN_310247600_345000_CN_310247604_345000/RConn1
  T_310247604__/LConn2 -- _CN_310247600_345000_CN_310247604_345000/RConn2
  _CN_310247600_345000_CN_310247604_345000/RConn3 -- T_310247604__/LConn3 -- bus84/LConn1
  T_310421666_345000_신시흥_(Sin_Siheung)/LConn1 -- _CN_310421666_345000_CN_308711344_345000/LConn1
  T_310421666_345000_신시흥_(Sin_Siheung)/LConn2 -- _CN_310421666_345000_CN_308711344_345000/LConn2
  _CN_310421666_345000_CN_308711344_345000/LConn3 -- T_310421666_345000_신시흥_(Sin_Siheung)/LConn3 -- bus85/LConn1
  T_308711344_345000_서서울_(Seo_Seoul)/LConn1 -- _CN_310421666_345000_CN_308711344_345000/RConn1
  T_308711344_345000_서서울_(Seo_Seoul)/LConn2 -- _CN_310421666_345000_CN_308711344_345000/RConn2
  _CN_310421666_345000_CN_308711344_345000/RConn3 -- T_308711344_345000_서서울_(Seo_Seoul)/LConn3 -- bus86/LConn1
  T_310293553_345000_/LConn1 -- _CN_310293553_345000_CN_310226153_345000/LConn1
  T_310293553_345000_/LConn2 -- _CN_310293553_345000_CN_310226153_345000/LConn2
  _CN_310293553_345000_CN_310226153_345000/LConn3 -- T_310293553_345000_/LConn3 -- bus87/LConn1
  _CN_310293553_345000_CN_310226153_345000/RConn1 -- T_310226153__신남원_(Sin_Namwon)/LConn1 -- _CN_310226151_345000_CN_310226153_345000/LConn1 -- _CN_310226153_345000_CN_387266330_345000/LConn1 -- _CN_310266398_345000_CN_310226153_345000/LConn1
  _CN_310293553_345000_CN_310226153_345000/RConn2 -- T_310226153__신남원_(Sin_Namwon)/LConn2 -- _CN_310226151_345000_CN_310226153_345000/LConn2 -- _CN_310226153_345000_CN_387266330_345000/LConn2 -- _CN_310266398_345000_CN_310226153_345000/LConn2
  _CN_310293553_345000_CN_310226153_345000/RConn3 -- T_310226153__신남원_(Sin_Namwon)/LConn3 -- _CN_310226151_345000_CN_310226153_345000/LConn3 -- _CN_310226153_345000_CN_387266330_345000/LConn3 -- bus88/LConn1 -- _CN_310266398_345000_CN_310226153_345000/LConn3
  T_311144491_345000_/LConn1 -- _CN_311144491_345000_CN_310226151_345000/LConn1
  T_311144491_345000_/LConn2 -- _CN_311144491_345000_CN_310226151_345000/LConn2
  _CN_311144491_345000_CN_310226151_345000/LConn3 -- T_311144491_345000_/LConn3 -- bus89/LConn1
  _CN_311144491_345000_CN_310226151_345000/RConn1 -- T_310226151_345000_신광주_(Sin_Gwangju)/LConn1 -- _CN_310226151_345000_CN_387266330_345000/LConn1 -- _CN_310226151_345000_CN_310226153_345000/RConn1
  _CN_311144491_345000_CN_310226151_345000/RConn2 -- T_310226151_345000_신광주_(Sin_Gwangju)/LConn2 -- _CN_310226151_345000_CN_387266330_345000/LConn2 -- _CN_310226151_345000_CN_310226153_345000/RConn2
  _CN_311144491_345000_CN_310226151_345000/RConn3 -- T_310226151_345000_신광주_(Sin_Gwangju)/LConn3 -- _CN_310226151_345000_CN_387266330_345000/LConn3 -- bus90/LConn1 -- _CN_310226151_345000_CN_310226153_345000/RConn3
  _CN_119001902_345000_CN_113679419_345000/LConn1 -- T_119001902_345000_청양_(Cheongyang)/LConn1 -- _CN_119001902_345000_CN_156580308_345000/RConn1
  _CN_119001902_345000_CN_113679419_345000/LConn2 -- T_119001902_345000_청양_(Cheongyang)/LConn2 -- _CN_119001902_345000_CN_156580308_345000/RConn2
  _CN_119001902_345000_CN_113679419_345000/LConn3 -- T_119001902_345000_청양_(Cheongyang)/LConn3 -- _CN_119001902_345000_CN_156580308_345000/RConn3 -- bus91/LConn1
  G_113679419_/RConn1 -- _CN_119001902_345000_CN_113679419_345000/RConn1
  G_113679419_/RConn2 -- _CN_119001902_345000_CN_113679419_345000/RConn2
  _CN_119001902_345000_CN_113679419_345000/RConn3 -- G_113679419_/RConn3 -- bus92/LConn1
  _CN_310266398_345000_CN_310226153_345000/RConn1 -- T_310266398_345000_/LConn1 -- _CN_310266398_345000_CN_310266400_345000/RConn1 -- _CN_310266398_345000_CN_308786013_345000/LConn1 -- _CN_310266398_345000_CN_308770040_345000/LConn1
  _CN_310266398_345000_CN_310226153_345000/RConn2 -- T_310266398_345000_/LConn2 -- _CN_310266398_345000_CN_310266400_345000/RConn2 -- _CN_310266398_345000_CN_308786013_345000/LConn2 -- _CN_310266398_345000_CN_308770040_345000/LConn2
  _CN_310266398_345000_CN_310226153_345000/RConn3 -- T_310266398_345000_/LConn3 -- _CN_310266398_345000_CN_310266400_345000/RConn3 -- bus93/LConn1 -- _CN_310266398_345000_CN_308786013_345000/LConn3 -- _CN_310266398_345000_CN_308770040_345000/LConn3
  T_308786013_345000_서대구_(Seo_Daegu)/LConn1 -- _CN_310266398_345000_CN_308786013_345000/RConn1
  T_308786013_345000_서대구_(Seo_Daegu)/LConn2 -- _CN_310266398_345000_CN_308786013_345000/RConn2
  _CN_310266398_345000_CN_308786013_345000/RConn3 -- T_308786013_345000_서대구_(Seo_Daegu)/LConn3 -- bus94/LConn1
  T_308770040__고령_(Goryeong)/LConn1 -- _CN_310266398_345000_CN_308770040_345000/RConn1
  T_308770040__고령_(Goryeong)/LConn2 -- _CN_310266398_345000_CN_308770040_345000/RConn2
  _CN_310266398_345000_CN_308770040_345000/RConn3 -- T_308770040__고령_(Goryeong)/LConn3 -- bus95/LConn1
  T_310421552__/LConn1 -- _CN_307934520_345000_CN_310421552_345000/RConn1
  T_310421552__/LConn2 -- _CN_307934520_345000_CN_310421552_345000/RConn2
  _CN_307934520_345000_CN_310421552_345000/RConn3 -- T_310421552__/LConn3 -- bus96/LConn1
  T_311223101_345000_동해_(Donghae)/LConn1 -- _CN_311223101_345000_CN_277786990_345000/LConn1
  T_311223101_345000_동해_(Donghae)/LConn2 -- _CN_311223101_345000_CN_277786990_345000/LConn2
  _CN_311223101_345000_CN_277786990_345000/LConn3 -- T_311223101_345000_동해_(Donghae)/LConn3 -- bus97/LConn1
  _CN_311223101_345000_CN_277786990_345000/RConn1 -- G_277786990_/RConn1 -- _CN_310995902_345000_CN_277786990_345000/LConn1
  _CN_311223101_345000_CN_277786990_345000/RConn2 -- G_277786990_/RConn2 -- _CN_310995902_345000_CN_277786990_345000/LConn2
  _CN_311223101_345000_CN_277786990_345000/RConn3 -- G_277786990_/RConn3 -- _CN_310995902_345000_CN_277786990_345000/LConn3 -- bus98/LConn1
  _CN_310995902_345000_CN_277786990_345000/RConn1 -- T_310995902_345000_신영주_(Sin_Yeongju)/LConn1 -- _CN_310995902_345000_CN_143605191_345000/RConn1
  _CN_310995902_345000_CN_277786990_345000/RConn2 -- T_310995902_345000_신영주_(Sin_Yeongju)/LConn2 -- _CN_310995902_345000_CN_143605191_345000/RConn2
  _CN_310995902_345000_CN_277786990_345000/RConn3 -- T_310995902_345000_신영주_(Sin_Yeongju)/LConn3 -- _CN_310995902_345000_CN_143605191_345000/RConn3 -- bus99/LConn1
  _CN_310961238_345000_CN_310963709_345000/RConn1 -- T_310963709__양주_(Yangju)/LConn1 -- _CN_312297594_345000_CN_310963709_345000/LConn1
  _CN_310961238_345000_CN_310963709_345000/RConn2 -- T_310963709__양주_(Yangju)/LConn2 -- _CN_312297594_345000_CN_310963709_345000/LConn2
  _CN_310961238_345000_CN_310963709_345000/RConn3 -- T_310963709__양주_(Yangju)/LConn3 -- _CN_312297594_345000_CN_310963709_345000/LConn3 -- bus100/LConn1
  _CN_310226151_345000_CN_387266330_345000/RConn1 -- G_387266330_Yeonggwang_Nuclear_Power_Plant/RConn1 -- _CN_310226153_345000_CN_387266330_345000/RConn1
  _CN_310226151_345000_CN_387266330_345000/RConn2 -- G_387266330_Yeonggwang_Nuclear_Power_Plant/RConn2 -- _CN_310226153_345000_CN_387266330_345000/RConn2
  _CN_310226151_345000_CN_387266330_345000/RConn3 -- G_387266330_Yeonggwang_Nuclear_Power_Plant/RConn3 -- _CN_310226153_345000_CN_387266330_345000/RConn3 -- bus101/LConn1
  G_313247875_/RConn1 -- _CN_308953834_345000_CN_313247875_345000/RConn1
  G_313247875_/RConn2 -- _CN_308953834_345000_CN_313247875_345000/RConn2
  _CN_308953834_345000_CN_313247875_345000/RConn3 -- G_313247875_/RConn3 -- bus102/LConn1
  _CN_312297594_345000_CN_235152926_345000/LConn1 -- T_312297594_345000_신파주_(Sin_Paju)/LConn1 -- _CN_312297594_345000_CN_310963709_345000/RConn1
  _CN_312297594_345000_CN_235152926_345000/LConn2 -- T_312297594_345000_신파주_(Sin_Paju)/LConn2 -- _CN_312297594_345000_CN_310963709_345000/RConn2
  _CN_312297594_345000_CN_235152926_345000/LConn3 -- T_312297594_345000_신파주_(Sin_Paju)/LConn3 -- _CN_312297594_345000_CN_310963709_345000/RConn3 -- bus103/LConn1
  G_235152926_인천화력발전소/RConn1 -- _CN_312297594_345000_CN_235152926_345000/RConn1
  G_235152926_인천화력발전소/RConn2 -- _CN_312297594_345000_CN_235152926_345000/RConn2
  _CN_312297594_345000_CN_235152926_345000/RConn3 -- G_235152926_인천화력발전소/RConn3 -- bus104/LConn1
  T_172009221_154000_/RConn1 -- L_172009221/LConn1
  T_172009221_154000_/RConn2 -- L_172009221/LConn2
  L_172009221/LConn3 -- T_172009221_154000_/RConn3 -- bus105/LConn1
  T_119180549__/RConn1 -- L_119180549/LConn1
  T_119180549__/RConn2 -- L_119180549/LConn2
  L_119180549/LConn3 -- T_119180549__/RConn3 -- bus106/LConn1
  T_312375473_154000_/RConn1 -- L_312375473/LConn1
  T_312375473_154000_/RConn2 -- L_312375473/LConn2
  L_312375473/LConn3 -- T_312375473_154000_/RConn3 -- bus107/LConn1
  T_313654649_154000_/RConn1 -- L_313654649/LConn1
  T_313654649_154000_/RConn2 -- L_313654649/LConn2
  L_313654649/LConn3 -- T_313654649_154000_/RConn3 -- bus108/LConn1
  T_180075042_154000_/RConn1 -- L_180075042/LConn1
  T_180075042_154000_/RConn2 -- L_180075042/LConn2
  L_180075042/LConn3 -- T_180075042_154000_/RConn3 -- bus109/LConn1
  T_168904645__양양변전소/RConn1 -- L_168904645/LConn1
  T_168904645__양양변전소/RConn2 -- L_168904645/LConn2
  L_168904645/LConn3 -- T_168904645__양양변전소/RConn3 -- bus110/LConn1
  T_313283373_154000_/RConn1 -- L_313283373/LConn1
  T_313283373_154000_/RConn2 -- L_313283373/LConn2
  L_313283373/LConn3 -- T_313283373_154000_/RConn3 -- bus111/LConn1
  T_311068711_154000_/RConn1 -- L_311068711/LConn1
  T_311068711_154000_/RConn2 -- L_311068711/LConn2
  L_311068711/LConn3 -- T_311068711_154000_/RConn3 -- bus112/LConn1
  T_205296347__/RConn1 -- L_205296347/LConn1
  T_205296347__/RConn2 -- L_205296347/LConn2
  L_205296347/LConn3 -- T_205296347__/RConn3 -- bus113/LConn1
  T_311144496_154000_/RConn1 -- L_311144496/LConn1
  T_311144496_154000_/RConn2 -- L_311144496/LConn2
  L_311144496/LConn3 -- T_311144496_154000_/RConn3 -- bus114/LConn1
  T_316124722_154000_/RConn1 -- L_316124722/LConn1
  T_316124722_154000_/RConn2 -- L_316124722/LConn2
  L_316124722/LConn3 -- T_316124722_154000_/RConn3 -- bus115/LConn1
  T_313388404_154000_/RConn1 -- L_313388404/LConn1
  T_313388404_154000_/RConn2 -- L_313388404/LConn2
  L_313388404/LConn3 -- T_313388404_154000_/RConn3 -- bus116/LConn1
  T_125840986__/RConn1 -- L_125840986/LConn1
  T_125840986__/RConn2 -- L_125840986/LConn2
  L_125840986/LConn3 -- T_125840986__/RConn3 -- bus117/LConn1
  T_126047655__/RConn1 -- L_126047655/LConn1
  T_126047655__/RConn2 -- L_126047655/LConn2
  L_126047655/LConn3 -- T_126047655__/RConn3 -- bus118/LConn1
  T_231045732__/RConn1 -- L_231045732/LConn1
  T_231045732__/RConn2 -- L_231045732/LConn2
  L_231045732/LConn3 -- T_231045732__/RConn3 -- bus119/LConn1
  T_312297600_154000_/RConn1 -- L_312297600/LConn1
  T_312297600_154000_/RConn2 -- L_312297600/LConn2
  L_312297600/LConn3 -- T_312297600_154000_/RConn3 -- bus120/LConn1
  T_313247877_154000_/RConn1 -- L_313247877/LConn1
  T_313247877_154000_/RConn2 -- L_313247877/LConn2
  L_313247877/LConn3 -- T_313247877_154000_/RConn3 -- bus121/LConn1
  T_313264823_154000_/RConn1 -- L_313264823/LConn1
  T_313264823_154000_/RConn2 -- L_313264823/LConn2
  L_313264823/LConn3 -- T_313264823_154000_/RConn3 -- bus122/LConn1
  T_297601178_154000_/RConn1 -- L_297601178/LConn1
  T_297601178_154000_/RConn2 -- L_297601178/LConn2
  L_297601178/LConn3 -- T_297601178_154000_/RConn3 -- bus123/LConn1
  T_297601183_154000_/RConn1 -- L_297601183/LConn1
  T_297601183_154000_/RConn2 -- L_297601183/LConn2
  L_297601183/LConn3 -- T_297601183_154000_/RConn3 -- bus124/LConn1
  T_308765054_345000_/RConn1 -- L_308765054/LConn1
  T_308765054_345000_/RConn2 -- L_308765054/LConn2
  L_308765054/LConn3 -- T_308765054_345000_/RConn3 -- bus125/LConn1
  T_313280968_154000_/RConn1 -- L_313280968/LConn1
  T_313280968_154000_/RConn2 -- L_313280968/LConn2
  L_313280968/LConn3 -- T_313280968_154000_/RConn3 -- bus126/LConn1
  T_312319437_154000_/RConn1 -- L_312319437/LConn1
  T_312319437_154000_/RConn2 -- L_312319437/LConn2
  L_312319437/LConn3 -- T_312319437_154000_/RConn3 -- bus127/LConn1
  T_312319401__/RConn1 -- L_312319401/LConn1
  T_312319401__/RConn2 -- L_312319401/LConn2
  L_312319401/LConn3 -- T_312319401__/RConn3 -- bus128/LConn1
  T_312319351_154000_/RConn1 -- L_312319351/LConn1
  T_312319351_154000_/RConn2 -- L_312319351/LConn2
  L_312319351/LConn3 -- T_312319351_154000_/RConn3 -- bus129/LConn1
  T_312375513_154000_/RConn1 -- L_312375513/LConn1
  T_312375513_154000_/RConn2 -- L_312375513/LConn2
  L_312375513/LConn3 -- T_312375513_154000_/RConn3 -- bus130/LConn1
  T_312375502_154000_/RConn1 -- L_312375502/LConn1
  T_312375502_154000_/RConn2 -- L_312375502/LConn2
  L_312375502/LConn3 -- T_312375502_154000_/RConn3 -- bus131/LConn1
  T_313264824_154000_/RConn1 -- L_313264824/LConn1
  T_313264824_154000_/RConn2 -- L_313264824/LConn2
  L_313264824/LConn3 -- T_313264824_154000_/RConn3 -- bus132/LConn1
  T_308953870__신진천_(Sin_Jincheon)/RConn1 -- L_308953870/LConn1
  T_308953870__신진천_(Sin_Jincheon)/RConn2 -- L_308953870/LConn2
  L_308953870/LConn3 -- T_308953870__신진천_(Sin_Jincheon)/RConn3 -- bus133/LConn1
  T_371952375__/RConn1 -- L_371952375/LConn1
  T_371952375__/RConn2 -- L_371952375/LConn2
  L_371952375/LConn3 -- T_371952375__/RConn3 -- bus134/LConn1
  T_372869919_154000_/RConn1 -- L_372869919/LConn1
  T_372869919_154000_/RConn2 -- L_372869919/LConn2
  L_372869919/LConn3 -- T_372869919_154000_/RConn3 -- bus135/LConn1
  T_312375499_154000_/RConn1 -- L_312375499/LConn1
  T_312375499_154000_/RConn2 -- L_312375499/LConn2
  L_312375499/LConn3 -- T_312375499_154000_/RConn3 -- bus136/LConn1
  T_312375501_154000_/RConn1 -- L_312375501/LConn1
  T_312375501_154000_/RConn2 -- L_312375501/LConn2
  L_312375501/LConn3 -- T_312375501_154000_/RConn3 -- bus137/LConn1
  T_310395601_154000_/RConn1 -- L_310395601/LConn1
  T_310395601_154000_/RConn2 -- L_310395601/LConn2
  L_310395601/LConn3 -- T_310395601_154000_/RConn3 -- bus138/LConn1
  T_310395617_154000_/RConn1 -- L_310395617/LConn1
  T_310395617_154000_/RConn2 -- L_310395617/LConn2
  L_310395617/LConn3 -- T_310395617_154000_/RConn3 -- bus139/LConn1
  T_312375515_154000_/RConn1 -- L_312375515/LConn1
  T_312375515_154000_/RConn2 -- L_312375515/LConn2
  L_312375515/LConn3 -- T_312375515_154000_/RConn3 -- bus140/LConn1
  T_312424737_154000_/RConn1 -- L_312424737/LConn1
  T_312424737_154000_/RConn2 -- L_312424737/LConn2
  L_312424737/LConn3 -- T_312424737_154000_/RConn3 -- bus141/LConn1
  T_312424733_154000_/RConn1 -- L_312424733/LConn1
  T_312424733_154000_/RConn2 -- L_312424733/LConn2
  L_312424733/LConn3 -- T_312424733_154000_/RConn3 -- bus142/LConn1
  T_312424741_154000_/RConn1 -- L_312424741/LConn1
  T_312424741_154000_/RConn2 -- L_312424741/LConn2
  L_312424741/LConn3 -- T_312424741_154000_/RConn3 -- bus143/LConn1
  T_313355100_154000_/RConn1 -- L_313355100/LConn1
  T_313355100_154000_/RConn2 -- L_313355100/LConn2
  L_313355100/LConn3 -- T_313355100_154000_/RConn3 -- bus144/LConn1
  T_313355118_154000_/RConn1 -- L_313355118/LConn1
  T_313355118_154000_/RConn2 -- L_313355118/LConn2
  L_313355118/LConn3 -- T_313355118_154000_/RConn3 -- bus145/LConn1
  T_313355123_154000_/RConn1 -- L_313355123/LConn1
  T_313355123_154000_/RConn2 -- L_313355123/LConn2
  L_313355123/LConn3 -- T_313355123_154000_/RConn3 -- bus146/LConn1
  T_313388489_154000_/RConn1 -- L_313388489/LConn1
  T_313388489_154000_/RConn2 -- L_313388489/LConn2
  L_313388489/LConn3 -- T_313388489_154000_/RConn3 -- bus147/LConn1
  T_312408983_154000_/RConn1 -- L_312408983/LConn1
  T_312408983_154000_/RConn2 -- L_312408983/LConn2
  L_312408983/LConn3 -- T_312408983_154000_/RConn3 -- bus148/LConn1
  T_415837596__/RConn1 -- L_415837596/LConn1
  T_415837596__/RConn2 -- L_415837596/LConn2
  L_415837596/LConn3 -- T_415837596__/RConn3 -- bus149/LConn1
  T_312319393_154000_/RConn1 -- L_312319393/LConn1
  T_312319393_154000_/RConn2 -- L_312319393/LConn2
  L_312319393/LConn3 -- T_312319393_154000_/RConn3 -- bus150/LConn1
  T_308953834_345000_/RConn1 -- L_308953834/LConn1
  T_308953834_345000_/RConn2 -- L_308953834/LConn2
  L_308953834/LConn3 -- T_308953834_345000_/RConn3 -- bus151/LConn1
  T_310574466_345000_/RConn1 -- L_310574466/LConn1
  T_310574466_345000_/RConn2 -- L_310574466/LConn2
  L_310574466/LConn3 -- T_310574466_345000_/RConn3 -- bus152/LConn1
  T_143756950_345000_/RConn1 -- L_143756950/LConn1
  T_143756950_345000_/RConn2 -- L_143756950/LConn2
  L_143756950/LConn3 -- T_143756950_345000_/RConn3 -- bus153/LConn1
  T_117614725__/RConn1 -- L_117614725/LConn1
  T_117614725__/RConn2 -- L_117614725/LConn2
  L_117614725/LConn3 -- T_117614725__/RConn3 -- bus154/LConn1
  T_310281736_345000_/RConn1 -- L_310281736/LConn1
  T_310281736_345000_/RConn2 -- L_310281736/LConn2
  L_310281736/LConn3 -- T_310281736_345000_/RConn3 -- bus155/LConn1
  T_143987473_345000_/RConn1 -- L_143987473/LConn1
  T_143987473_345000_/RConn2 -- L_143987473/LConn2
  L_143987473/LConn3 -- T_143987473_345000_/RConn3 -- bus156/LConn1
  T_310943500_345000_동서울_변전소/RConn1 -- L_310943500/LConn1
  T_310943500_345000_동서울_변전소/RConn2 -- L_310943500/LConn2
  L_310943500/LConn3 -- T_310943500_345000_동서울_변전소/RConn3 -- bus157/LConn1
  T_310961238_345000_/RConn1 -- L_310961238/LConn1
  T_310961238_345000_/RConn2 -- L_310961238/LConn2
  L_310961238/LConn3 -- T_310961238_345000_/RConn3 -- bus158/LConn1
  T_143605191_345000_신포항_(Sin_Pohang)/RConn1 -- L_143605191/LConn1
  T_143605191_345000_신포항_(Sin_Pohang)/RConn2 -- L_143605191/LConn2
  L_143605191/LConn3 -- T_143605191_345000_신포항_(Sin_Pohang)/RConn3 -- bus159/LConn1
  T_308733209_345000_/RConn1 -- L_308733209/LConn1
  T_308733209_345000_/RConn2 -- L_308733209/LConn2
  L_308733209/LConn3 -- T_308733209_345000_/RConn3 -- bus160/LConn1
  T_310247600_345000_/RConn1 -- L_310247600/LConn1
  T_310247600_345000_/RConn2 -- L_310247600/LConn2
  L_310247600/LConn3 -- T_310247600_345000_/RConn3 -- bus161/LConn1
  T_308733211__/RConn1 -- L_308733211/LConn1
  T_308733211__/RConn2 -- L_308733211/LConn2
  L_308733211/LConn3 -- T_308733211__/RConn3 -- bus162/LConn1
  T_198717854__/RConn1 -- L_198717854/LConn1
  T_198717854__/RConn2 -- L_198717854/LConn2
  L_198717854/LConn3 -- T_198717854__/RConn3 -- bus163/LConn1
  T_307934520__/RConn1 -- L_307934520/LConn1
  T_307934520__/RConn2 -- L_307934520/LConn2
  L_307934520/LConn3 -- T_307934520__/RConn3 -- bus164/LConn1
  T_199954117__/RConn1 -- L_199954117/LConn1
  T_199954117__/RConn2 -- L_199954117/LConn2
  L_199954117/LConn3 -- T_199954117__/RConn3 -- bus165/LConn1
  T_156580308_345000_신옥천_(Sin_Okcheon)/RConn1 -- L_156580308/LConn1
  T_156580308_345000_신옥천_(Sin_Okcheon)/RConn2 -- L_156580308/LConn2
  L_156580308/LConn3 -- T_156580308_345000_신옥천_(Sin_Okcheon)/RConn3 -- bus166/LConn1
  T_310247604__/RConn1 -- L_310247604/LConn1
  T_310247604__/RConn2 -- L_310247604/LConn2
  L_310247604/LConn3 -- T_310247604__/RConn3 -- bus167/LConn1
  T_310421666_345000_신시흥_(Sin_Siheung)/RConn1 -- L_310421666/LConn1
  T_310421666_345000_신시흥_(Sin_Siheung)/RConn2 -- L_310421666/LConn2
  L_310421666/LConn3 -- T_310421666_345000_신시흥_(Sin_Siheung)/RConn3 -- bus168/LConn1
  T_310226153__신남원_(Sin_Namwon)/RConn1 -- L_310226153/LConn1
  T_310226153__신남원_(Sin_Namwon)/RConn2 -- L_310226153/LConn2
  L_310226153/LConn3 -- T_310226153__신남원_(Sin_Namwon)/RConn3 -- bus169/LConn1
  T_311144491_345000_/RConn1 -- L_311144491/LConn1
  T_311144491_345000_/RConn2 -- L_311144491/LConn2
  L_311144491/LConn3 -- T_311144491_345000_/RConn3 -- bus170/LConn1
  T_119001902_345000_청양_(Cheongyang)/RConn1 -- L_119001902/LConn1
  T_119001902_345000_청양_(Cheongyang)/RConn2 -- L_119001902/LConn2
  L_119001902/LConn3 -- T_119001902_345000_청양_(Cheongyang)/RConn3 -- bus171/LConn1
  T_310266398_345000_/RConn1 -- L_310266398/LConn1
  T_310266398_345000_/RConn2 -- L_310266398/LConn2
  L_310266398/LConn3 -- T_310266398_345000_/RConn3 -- bus172/LConn1
  T_308786013_345000_서대구_(Seo_Daegu)/RConn1 -- L_308786013/LConn1
  T_308786013_345000_서대구_(Seo_Daegu)/RConn2 -- L_308786013/LConn2
  L_308786013/LConn3 -- T_308786013_345000_서대구_(Seo_Daegu)/RConn3 -- bus173/LConn1
  T_311223101_345000_동해_(Donghae)/RConn1 -- L_311223101/LConn1
  T_311223101_345000_동해_(Donghae)/RConn2 -- L_311223101/LConn2
  L_311223101/LConn3 -- T_311223101_345000_동해_(Donghae)/RConn3 -- bus174/LConn1
  T_310995902_345000_신영주_(Sin_Yeongju)/RConn1 -- L_310995902/LConn1
  T_310995902_345000_신영주_(Sin_Yeongju)/RConn2 -- L_310995902/LConn2
  L_310995902/LConn3 -- T_310995902_345000_신영주_(Sin_Yeongju)/RConn3 -- bus175/LConn1
